simulink model "Drone2_simulink_old1"  (R2024b)
settings: Solver=ode1be  StartTime=0.0  StopTime=1200  FixedStep=0.001  MaxStep=0.001  MinStep=0.00095  RelTol=1e-3
undefined symbols (not defined in the file): DiscIntNeverNeededParam, Environment, Newton, Raphson, Sim3dSensor, Vehicle, X, Y, Z
libraries: sm_lib x2951, nesl_utility x76, slpidlib x25, simulink x4, eeGeneralControl x4, matrix_library x3, rllib x2, sim3dlib x2, uavsim3dlib x2, dspstat3 x1, SignalEditorBlockLib x1, sharedutil x1
(part 3 of 21)

== system Drone2_simulink_old1/Controller/RL System ==
  In1 : Inport
  In2 : Inport  Port=2
  In3 : Inport  Port=3
  In4 : Inport  Port=4
  In5 : Inport  Port=5
  In6 : Inport  Port=6
  In7 : Inport  Port=7
  In8 : Inport  Port=8
  In9 : Inport  Port=9
  In10 : Inport  Port=10
  isdone : Inport  Port=11
  Constant10 : Constant  Commented=on  Value=-4
  Constant11 : Constant  Commented=on  Value=0
  Demux : Demux  Commented=on  Outputs=2
  MATLAB Function2 : MATLAB Function  Commented=on  TreatAsAtomicUnit=on
  MATLAB Function3 : MATLAB Function  Commented=on  TreatAsAtomicUnit=on  mask{MaxPose=Vehicle.Syringe.Front.maxpos, MinPose=Vehicle.Syringe.Front.minpos, MaxVel=Vehicle.Syringe.MaxVelocity, Delta=0.0050, K=500.0}
  MATLAB Function4 : MATLAB Function  Commented=on  TreatAsAtomicUnit=on  mask{MaxPose=Vehicle.Syringe.Front.maxpos, MinPose=Vehicle.Syringe.Front.minpos, MaxVel=Vehicle.Syringe.MaxVelocity, Delta=0.0050}
  Mux : Mux  Commented=on  Inputs=2
  Mux1 : Mux  Commented=on  Inputs=12
  RL Agent : rllib/RL Agent  Commented=on  Agent=Controller.agent  ExternalActionAsInput=off  ProvideLastAction=off  ProvideCumRwd=off  TreatAsDirectFeedthrough=on  UseStrictObservationDataTypes=off
  Reshape : Reshape  Commented=on  OutputDimensionality=Customize
  front : Outport
  Back : Outport  Port=2
  wires:
  Mux1/1 -> MATLAB Function4/1(obs), RL Agent/1
  Constant10/1 -> Mux1/11, Mux/1
  Mux/1 -> MATLAB Function4/2(desired)
  In6/1 -> Mux1/6
  MATLAB Function4/1(reward) -> Reshape/1
  Constant11/1 -> Mux1/12, Mux/2
  In5/1 -> Mux1/5
  Reshape/1 -> RL Agent/2
  RL Agent/1 -> Demux/1
  In10/1 -> Mux1/10
  In4/1 -> Mux1/4
  In2/1 -> Mux1/2
  In3/1 -> Mux1/3
  isdone/1 -> RL Agent/3
  In7/1 -> Mux1/7
  In8/1 -> Mux1/8
  In9/1 -> Mux1/9
  Demux/1 -> front/1
  Demux/2 -> Back/1
  In1/1 -> Mux1/1

== system Drone2_simulink_old1/Controller/Underwater_Syringe_Actuation ==
  Z : Inport
  Z_desired : Inport  Port=2
  Vf_1 : Inport  Port=3
  Vf_2 : Inport  Port=4
  Theta : Inport  Port=5
  Theta Desired : Inport  Port=6
  Vb_prev : Inport  Port=7
  Derivative : Derivative  Commented=on
  Derivative1 : Derivative
  Discrete Derivative : simulink/Discrete/Discrete Derivative  Commented=on  gainval=1.0  ICPrevScaledInput=0.0  OutMin=[]  OutMax=[]  OutDataType=fixdt(1, 16)  OutScaling=2^-10  DoSatur=off
  Gain4 : Gain  Gain=0.5
  MATLAB Function1 : MATLAB Function  Commented=on  TreatAsAtomicUnit=on  mask{V_MIN=Vehicle.Syringe.Front.minpos, V_MAX=Vehicle.Syringe.Front.maxpos, V_DOT_MAX=0.012, HF=0.2, A=0, g=9.81, rho=1000, dt=0.001, Kp_pos=0.002, Kp_vel=0.002, Kr=0.005, EZDB=0.05, sigma=0.1, Ez_high=1, PLRate=0.0002, PKRate=0.05, ETDB=3}
      mask prompts: V_MIN "Min"; V_MAX "Max"; V_DOT_MAX "max rate"; HF "Half Length of drone"; A "Area of Syringe"; g "Gravity"; rho "Density"; dt "Sample Time"; Kp_pos "Learning Rate-Pose"; Kp_vel "Slow Learning Rate"; Kr "K_Rate"; EZDB "Error zone to reduce adaption"; sigma "Steady state error region"; Ez_high "mode switch region"; PLRate "Pitch Learning Rate"; PKRate "K_Rate"; ETDB "Error zone to reduce adaption"
  MATLAB Function7 : MATLAB Function  TreatAsAtomicUnit=on  mask{Min=Vehicle.Syringe.Front.minpos, Max=Vehicle.Syringe.Front.maxpos, HF=0.2, AS=0, G=9.81, RHO=1000, DT=0.001, DFRate=0.02, DMRate=0.002, DSRate=0.002, Dpanelty=0.005, EZDB=0.05, PLRate=0.0002, PKRate=0.05, ETDB=3}
      mask prompts: HF "Half Length of drone"; AS "Area of Syringe"; G "Gravity"; RHO "Density"; DT "Sample Time"; DFRate "Fast Learning rate with |e|>1"; DMRate "Medium Learning Rate"; DSRate "Slow Learning Rate"; Dpanelty "K_Rate"; EZDB "Error zone to reduce adaption"; PLRate "Pitch Learning Rate"; PKRate "K_Rate"; ETDB "Error zone to reduce adaption"
  PID Controller1 : slpidlib/PID Controller  Commented=on  Controller=PD  Form=Parallel  TimeDomain=Continuous-time  UseExternalTs=off  SampleTime=-1  IntegratorMethod=Forward Euler  FilterMethod=Forward Euler  ControllerParametersSource=internal  P=3500.0200194669353  I=843.52365195509  UseKiTs=on  D=26.9299392102605  UseExternalDerivativeSource=off  N=0.579906738639273  UseFilter=on  TunerSelectOption=Transfer Function Based (PID Tuner App)  InitialConditionSource=internal  InitialConditionForIntegrator=0  InitialConditionForFilter=0  DifferentiatorICPrevScaledInput=0  ExternalReset=none  TrackingMode=off  Kt=1  LimitOutput=on  SatLimitsSource=internal  UpperSaturationLimit=40  LowerSaturationLimit=0  LinearizeAsGain=on  AntiWindupMode=none  Kb=1  LimitIntegrator=off  UpperIntegratorSaturationLimit=inf  LowerIntegratorSaturationLimit=-inf  POutMin=[]  POutMax=[]  IOutMin=[]  IOutMax=[]  DOutMin=[]  DOutMax=[]  NOutMin=[]  NOutMax=[]  SumOutMin=[]  SumOutMax=[]  SaturationOutMin=[]  SaturationOutMax=[]  PParamMin=[]  PParamMax=[]  IParamMin=[]  IParamMax=[]  DParamMin=[]  DParamMax=[]  NParamMin=[]  NParamMax=[]  KbParamMin=[]  KbParamMax=[]  KtParamMin=[]  KtParamMax=[]  KbOutMin=[]  KbOutMax=[]  KtOutMin=[]  KtOutMax=[]  IntegratorOutMin=[]  IntegratorOutMax=[]  FilterOutMin=[]  FilterOutMax=[]  SumI1OutMin=[]  SumI1OutMax=[]  SumI2OutMin=[]  SumI2OutMax=[]  SumI3OutMin=[]  SumI3OutMax=[]  SumI4OutMin=[]  SumI4OutMax=[]  SumDOutMin=[]  SumDOutMax=[]  DifferentiatorOutMin=[]  DifferentiatorOutMax=[]  FilterDiffOutCoefMin=[]  FilterDiffOutCoefMax=[]  ReciprocalOutMin=[]  ReciprocalOutMax=[]  SumDenOutMin=[]  SumDenOutMax=[]  SumNumOutMin=[]  SumNumOutMax=[]  DivideOutMin=[]  DivideOutMax=[]  UdiffTsProdOutMin=[]  UdiffTsProdOutMax=[]  NTsProdOutMin=[]  NTsProdOutMax=[]  UintegralTsProdOutMin=[]  UintegralTsProdOutMax=[]  UngainTsProdOutMin=[]  UngainTsProdOutMax=[]  ClampingZeroOutDataTypeStr=Inherit: Inherit via back propagation  ClampingZeroOutMin=[]  ClampingZeroOutMax=[]  FilterDenConstantOutDataTypeStr=Inherit: Inherit via back propagation  FilterDenConstantOutMin=[]  FilterDenConstantOutMax=[]  PCopyOutDataTypeStr=Inherit: Inherit via back propagation  PCopyOutMin=[]  PCopyOutMax=[]  NCopyOutDataTypeStr=Inherit: Inherit via back propagation  NCopyOutMin=[]  NCopyOutMax=[]  IntegratorContinuousStateAttributes=''  IntegratorStateMustResolveToSignalObject=off  IntegratorRTWStateStorageClass=Auto  FilterContinuousStateAttributes=''  FilterStateMustResolveToSignalObject=off  FilterRTWStateStorageClass=Auto  ParallelPVariant=InternalParameters  IdealPVariant=Disabled  IVariant=Disabled  DVariant=InternalParameters  IntegratorVariant=Disabled  SatVariant=Enabled  AWVariant=Disabled  PCopyVariant=Disabled  TRVariant=Disabled  FdbkBlocksVariant=Forward  IdealPFdbkVariant=Disabled  SatFdbkVariant=Disabled  DerivativeFilterVariant=ContFilter  NVariant=InternalParameters  NCopyVariant=Disabled  FilterICVariant=InternalICsFilter  IntegratorICVariant=Disabled  ExternalResetVariant=Disabled  TRSumVariant=Passthrough  SumFdbkVariant=Disabled  SumVariant=Sum_PD  TsampFilterVariant=InternalTs  TsampNgainVariant=Passthrough  TsampIntegralVariant=Disabled_SignalSpec  ExternalSaturationOutDataTypeStr=Inherit: Same as second input  DerivativeSourceVariant=ErrorSignal
  PID Controller2 : slpidlib/PID Controller  Commented=on  Controller=PD  Form=Parallel  TimeDomain=Continuous-time  UseExternalTs=off  SampleTime=-1  IntegratorMethod=Forward Euler  FilterMethod=Forward Euler  ControllerParametersSource=internal  P=3744.13110896654  I=964.677966952311  UseKiTs=on  D=30  UseExternalDerivativeSource=off  N=0.58  UseFilter=on  TunerSelectOption=Transfer Function Based (PID Tuner App)  InitialConditionSource=internal  InitialConditionForIntegrator=0  InitialConditionForFilter=0  DifferentiatorICPrevScaledInput=0  ExternalReset=none  TrackingMode=off  Kt=1  LimitOutput=on  SatLimitsSource=internal  UpperSaturationLimit=40  LowerSaturationLimit=0  LinearizeAsGain=on  AntiWindupMode=none  Kb=1  LimitIntegrator=off  UpperIntegratorSaturationLimit=inf  LowerIntegratorSaturationLimit=-inf  POutMin=[]  POutMax=[]  IOutMin=[]  IOutMax=[]  DOutMin=[]  DOutMax=[]  NOutMin=[]  NOutMax=[]  SumOutMin=[]  SumOutMax=[]  SaturationOutMin=[]  SaturationOutMax=[]  PParamMin=[]  PParamMax=[]  IParamMin=[]  IParamMax=[]  DParamMin=[]  DParamMax=[]  NParamMin=[]  NParamMax=[]  KbParamMin=[]  KbParamMax=[]  KtParamMin=[]  KtParamMax=[]  KbOutMin=[]  KbOutMax=[]  KtOutMin=[]  KtOutMax=[]  IntegratorOutMin=[]  IntegratorOutMax=[]  FilterOutMin=[]  FilterOutMax=[]  SumI1OutMin=[]  SumI1OutMax=[]  SumI2OutMin=[]  SumI2OutMax=[]  SumI3OutMin=[]  SumI3OutMax=[]  SumI4OutMin=[]  SumI4OutMax=[]  SumDOutMin=[]  SumDOutMax=[]  DifferentiatorOutMin=[]  DifferentiatorOutMax=[]  FilterDiffOutCoefMin=[]  FilterDiffOutCoefMax=[]  ReciprocalOutMin=[]  ReciprocalOutMax=[]  SumDenOutMin=[]  SumDenOutMax=[]  SumNumOutMin=[]  SumNumOutMax=[]  DivideOutMin=[]  DivideOutMax=[]  UdiffTsProdOutMin=[]  UdiffTsProdOutMax=[]  NTsProdOutMin=[]  NTsProdOutMax=[]  UintegralTsProdOutMin=[]  UintegralTsProdOutMax=[]  UngainTsProdOutMin=[]  UngainTsProdOutMax=[]  ClampingZeroOutDataTypeStr=Inherit: Inherit via back propagation  ClampingZeroOutMin=[]  ClampingZeroOutMax=[]  FilterDenConstantOutDataTypeStr=Inherit: Inherit via back propagation  FilterDenConstantOutMin=[]  FilterDenConstantOutMax=[]  PCopyOutDataTypeStr=Inherit: Inherit via back propagation  PCopyOutMin=[]  PCopyOutMax=[]  NCopyOutDataTypeStr=Inherit: Inherit via back propagation  NCopyOutMin=[]  NCopyOutMax=[]  IntegratorContinuousStateAttributes=''  IntegratorStateMustResolveToSignalObject=off  IntegratorRTWStateStorageClass=Auto  FilterContinuousStateAttributes=''  FilterStateMustResolveToSignalObject=off  FilterRTWStateStorageClass=Auto  ParallelPVariant=InternalParameters  IdealPVariant=Disabled  IVariant=Disabled  DVariant=InternalParameters  IntegratorVariant=Disabled  SatVariant=Enabled  AWVariant=Disabled  PCopyVariant=Disabled  TRVariant=Disabled  FdbkBlocksVariant=Forward  IdealPFdbkVariant=Disabled  SatFdbkVariant=Disabled  DerivativeFilterVariant=ContFilter  NVariant=InternalParameters  NCopyVariant=Disabled  FilterICVariant=InternalICsFilter  IntegratorICVariant=Disabled  ExternalResetVariant=Disabled  TRSumVariant=Passthrough  SumFdbkVariant=Disabled  SumVariant=Sum_PD  TsampFilterVariant=InternalTs  TsampNgainVariant=Passthrough  TsampIntegralVariant=Disabled_SignalSpec  ExternalSaturationOutDataTypeStr=Inherit: Same as second input  DerivativeSourceVariant=ErrorSignal
  PID Controller4 : slpidlib/PID Controller  Controller=PD  Form=Parallel  TimeDomain=Continuous-time  UseExternalTs=off  SampleTime=-1  IntegratorMethod=Forward Euler  FilterMethod=Forward Euler  ControllerParametersSource=internal  P=8  I=0  UseKiTs=on  D=0.5  UseExternalDerivativeSource=off  N=20  UseFilter=on  TunerSelectOption=Transfer Function Based (PID Tuner App)  InitialConditionSource=internal  InitialConditionForIntegrator=0  InitialConditionForFilter=0  DifferentiatorICPrevScaledInput=0  ExternalReset=none  TrackingMode=off  Kt=1  LimitOutput=off  SatLimitsSource=internal  UpperSaturationLimit=Vehicle.Syringe.Thrustlim  LowerSaturationLimit=-Vehicle.Syringe.Thrustlim  LinearizeAsGain=on  AntiWindupMode=none  Kb=1  LimitIntegrator=off  UpperIntegratorSaturationLimit=inf  LowerIntegratorSaturationLimit=-inf  POutMin=[]  POutMax=[]  IOutMin=[]  IOutMax=[]  DOutMin=[]  DOutMax=[]  NOutMin=[]  NOutMax=[]  SumOutMin=[]  SumOutMax=[]  SaturationOutMin=[]  SaturationOutMax=[]  PParamMin=[]  PParamMax=[]  IParamMin=[]  IParamMax=[]  DParamMin=[]  DParamMax=[]  NParamMin=[]  NParamMax=[]  KbParamMin=[]  KbParamMax=[]  KtParamMin=[]  KtParamMax=[]  KbOutMin=[]  KbOutMax=[]  KtOutMin=[]  KtOutMax=[]  IntegratorOutMin=[]  IntegratorOutMax=[]  FilterOutMin=[]  FilterOutMax=[]  SumI1OutMin=[]  SumI1OutMax=[]  SumI2OutMin=[]  SumI2OutMax=[]  SumI3OutMin=[]  SumI3OutMax=[]  SumI4OutMin=[]  SumI4OutMax=[]  SumDOutMin=[]  SumDOutMax=[]  DifferentiatorOutMin=[]  DifferentiatorOutMax=[]  FilterDiffOutCoefMin=[]  FilterDiffOutCoefMax=[]  ReciprocalOutMin=[]  ReciprocalOutMax=[]  SumDenOutMin=[]  SumDenOutMax=[]  SumNumOutMin=[]  SumNumOutMax=[]  DivideOutMin=[]  DivideOutMax=[]  UdiffTsProdOutMin=[]  UdiffTsProdOutMax=[]  NTsProdOutMin=[]  NTsProdOutMax=[]  UintegralTsProdOutMin=[]  UintegralTsProdOutMax=[]  UngainTsProdOutMin=[]  UngainTsProdOutMax=[]  ClampingZeroOutDataTypeStr=Inherit: Inherit via back propagation  ClampingZeroOutMin=[]  ClampingZeroOutMax=[]  FilterDenConstantOutDataTypeStr=Inherit: Inherit via back propagation  FilterDenConstantOutMin=[]  FilterDenConstantOutMax=[]  PCopyOutDataTypeStr=Inherit: Inherit via back propagation  PCopyOutMin=[]  PCopyOutMax=[]  NCopyOutDataTypeStr=Inherit: Inherit via back propagation  NCopyOutMin=[]  NCopyOutMax=[]  IntegratorContinuousStateAttributes=''  IntegratorStateMustResolveToSignalObject=off  IntegratorRTWStateStorageClass=Auto  FilterContinuousStateAttributes=''  FilterStateMustResolveToSignalObject=off  FilterRTWStateStorageClass=Auto  ParallelPVariant=InternalParameters  IdealPVariant=Disabled  IVariant=Disabled  DVariant=InternalParameters  IntegratorVariant=Disabled  SatVariant=Disabled  AWVariant=Disabled  PCopyVariant=Disabled  TRVariant=Disabled  FdbkBlocksVariant=Forward  IdealPFdbkVariant=Disabled  SatFdbkVariant=Disabled  DerivativeFilterVariant=ContFilter  NVariant=InternalParameters  NCopyVariant=Disabled  FilterICVariant=InternalICsFilter  IntegratorICVariant=Disabled  ExternalResetVariant=Disabled  TRSumVariant=Passthrough  SumFdbkVariant=Disabled  SumVariant=Sum_PD  TsampFilterVariant=InternalTs  TsampNgainVariant=Passthrough  TsampIntegralVariant=Disabled_SignalSpec  ExternalSaturationOutDataTypeStr=Inherit: Same as second input  DerivativeSourceVariant=ErrorSignal
  PID Controller5 : slpidlib/PID Controller  Controller=PD  Form=Parallel  TimeDomain=Continuous-time  UseExternalTs=off  SampleTime=-1  IntegratorMethod=Forward Euler  FilterMethod=Forward Euler  ControllerParametersSource=internal  P=4  I=0  UseKiTs=on  D=0.5  UseExternalDerivativeSource=off  N=100  UseFilter=on  TunerSelectOption=Transfer Function Based (PID Tuner App)  InitialConditionSource=internal  InitialConditionForIntegrator=0  InitialConditionForFilter=0  DifferentiatorICPrevScaledInput=0  ExternalReset=none  TrackingMode=off  Kt=1  LimitOutput=off  SatLimitsSource=internal  UpperSaturationLimit=Vehicle.Syringe.Thrustlim  LowerSaturationLimit=-Vehicle.Syringe.Thrustlim  LinearizeAsGain=on  AntiWindupMode=none  Kb=1  LimitIntegrator=off  UpperIntegratorSaturationLimit=inf  LowerIntegratorSaturationLimit=-inf  POutMin=[]  POutMax=[]  IOutMin=[]  IOutMax=[]  DOutMin=[]  DOutMax=[]  NOutMin=[]  NOutMax=[]  SumOutMin=[]  SumOutMax=[]  SaturationOutMin=[]  SaturationOutMax=[]  PParamMin=[]  PParamMax=[]  IParamMin=[]  IParamMax=[]  DParamMin=[]  DParamMax=[]  NParamMin=[]  NParamMax=[]  KbParamMin=[]  KbParamMax=[]  KtParamMin=[]  KtParamMax=[]  KbOutMin=[]  KbOutMax=[]  KtOutMin=[]  KtOutMax=[]  IntegratorOutMin=[]  IntegratorOutMax=[]  FilterOutMin=[]  FilterOutMax=[]  SumI1OutMin=[]  SumI1OutMax=[]  SumI2OutMin=[]  SumI2OutMax=[]  SumI3OutMin=[]  SumI3OutMax=[]  SumI4OutMin=[]  SumI4OutMax=[]  SumDOutMin=[]  SumDOutMax=[]  DifferentiatorOutMin=[]  DifferentiatorOutMax=[]  FilterDiffOutCoefMin=[]  FilterDiffOutCoefMax=[]  ReciprocalOutMin=[]  ReciprocalOutMax=[]  SumDenOutMin=[]  SumDenOutMax=[]  SumNumOutMin=[]  SumNumOutMax=[]  DivideOutMin=[]  DivideOutMax=[]  UdiffTsProdOutMin=[]  UdiffTsProdOutMax=[]  NTsProdOutMin=[]  NTsProdOutMax=[]  UintegralTsProdOutMin=[]  UintegralTsProdOutMax=[]  UngainTsProdOutMin=[]  UngainTsProdOutMax=[]  ClampingZeroOutDataTypeStr=Inherit: Inherit via back propagation  ClampingZeroOutMin=[]  ClampingZeroOutMax=[]  FilterDenConstantOutDataTypeStr=Inherit: Inherit via back propagation  FilterDenConstantOutMin=[]  FilterDenConstantOutMax=[]  PCopyOutDataTypeStr=Inherit: Inherit via back propagation  PCopyOutMin=[]  PCopyOutMax=[]  NCopyOutDataTypeStr=Inherit: Inherit via back propagation  NCopyOutMin=[]  NCopyOutMax=[]  IntegratorContinuousStateAttributes=''  IntegratorStateMustResolveToSignalObject=off  IntegratorRTWStateStorageClass=Auto  FilterContinuousStateAttributes=''  FilterStateMustResolveToSignalObject=off  FilterRTWStateStorageClass=Auto  ParallelPVariant=InternalParameters  IdealPVariant=Disabled  IVariant=Disabled  DVariant=InternalParameters  IntegratorVariant=Disabled  SatVariant=Disabled  AWVariant=Disabled  PCopyVariant=Disabled  TRVariant=Disabled  FdbkBlocksVariant=Forward  IdealPFdbkVariant=Disabled  SatFdbkVariant=Disabled  DerivativeFilterVariant=ContFilter  NVariant=InternalParameters  NCopyVariant=Disabled  FilterICVariant=InternalICsFilter  IntegratorICVariant=Disabled  ExternalResetVariant=Disabled  TRSumVariant=Passthrough  SumFdbkVariant=Disabled  SumVariant=Sum_PD  TsampFilterVariant=InternalTs  TsampNgainVariant=Passthrough  TsampIntegralVariant=Disabled_SignalSpec  ExternalSaturationOutDataTypeStr=Inherit: Same as second input  DerivativeSourceVariant=ErrorSignal
  PID Controller6 : slpidlib/PID Controller  Controller=PD  Form=Parallel  TimeDomain=Continuous-time  UseExternalTs=off  SampleTime=-1  IntegratorMethod=Forward Euler  FilterMethod=Forward Euler  ControllerParametersSource=internal  P=3500  I=843.52365195509  UseKiTs=on  D=30  UseExternalDerivativeSource=off  N=1  UseFilter=on  TunerSelectOption=Transfer Function Based (PID Tuner App)  InitialConditionSource=internal  InitialConditionForIntegrator=0  InitialConditionForFilter=0  DifferentiatorICPrevScaledInput=0  ExternalReset=none  TrackingMode=off  Kt=1  LimitOutput=on  SatLimitsSource=internal  UpperSaturationLimit=40  LowerSaturationLimit=0  LinearizeAsGain=on  AntiWindupMode=none  Kb=1  LimitIntegrator=off  UpperIntegratorSaturationLimit=inf  LowerIntegratorSaturationLimit=-inf  POutMin=[]  POutMax=[]  IOutMin=[]  IOutMax=[]  DOutMin=[]  DOutMax=[]  NOutMin=[]  NOutMax=[]  SumOutMin=[]  SumOutMax=[]  SaturationOutMin=[]  SaturationOutMax=[]  PParamMin=[]  PParamMax=[]  IParamMin=[]  IParamMax=[]  DParamMin=[]  DParamMax=[]  NParamMin=[]  NParamMax=[]  KbParamMin=[]  KbParamMax=[]  KtParamMin=[]  KtParamMax=[]  KbOutMin=[]  KbOutMax=[]  KtOutMin=[]  KtOutMax=[]  IntegratorOutMin=[]  IntegratorOutMax=[]  FilterOutMin=[]  FilterOutMax=[]  SumI1OutMin=[]  SumI1OutMax=[]  SumI2OutMin=[]  SumI2OutMax=[]  SumI3OutMin=[]  SumI3OutMax=[]  SumI4OutMin=[]  SumI4OutMax=[]  SumDOutMin=[]  SumDOutMax=[]  DifferentiatorOutMin=[]  DifferentiatorOutMax=[]  FilterDiffOutCoefMin=[]  FilterDiffOutCoefMax=[]  ReciprocalOutMin=[]  ReciprocalOutMax=[]  SumDenOutMin=[]  SumDenOutMax=[]  SumNumOutMin=[]  SumNumOutMax=[]  DivideOutMin=[]  DivideOutMax=[]  UdiffTsProdOutMin=[]  UdiffTsProdOutMax=[]  NTsProdOutMin=[]  NTsProdOutMax=[]  UintegralTsProdOutMin=[]  UintegralTsProdOutMax=[]  UngainTsProdOutMin=[]  UngainTsProdOutMax=[]  ClampingZeroOutDataTypeStr=Inherit: Inherit via back propagation  ClampingZeroOutMin=[]  ClampingZeroOutMax=[]  FilterDenConstantOutDataTypeStr=Inherit: Inherit via back propagation  FilterDenConstantOutMin=[]  FilterDenConstantOutMax=[]  PCopyOutDataTypeStr=Inherit: Inherit via back propagation  PCopyOutMin=[]  PCopyOutMax=[]  NCopyOutDataTypeStr=Inherit: Inherit via back propagation  NCopyOutMin=[]  NCopyOutMax=[]  IntegratorContinuousStateAttributes=''  IntegratorStateMustResolveToSignalObject=off  IntegratorRTWStateStorageClass=Auto  FilterContinuousStateAttributes=''  FilterStateMustResolveToSignalObject=off  FilterRTWStateStorageClass=Auto  ParallelPVariant=InternalParameters  IdealPVariant=Disabled  IVariant=Disabled  DVariant=InternalParameters  IntegratorVariant=Disabled  SatVariant=Enabled  AWVariant=Disabled  PCopyVariant=Disabled  TRVariant=Disabled  FdbkBlocksVariant=Forward  IdealPFdbkVariant=Disabled  SatFdbkVariant=Disabled  DerivativeFilterVariant=ContFilter  NVariant=InternalParameters  NCopyVariant=Disabled  FilterICVariant=InternalICsFilter  IntegratorICVariant=Disabled  ExternalResetVariant=Disabled  TRSumVariant=Passthrough  SumFdbkVariant=Disabled  SumVariant=Sum_PD  TsampFilterVariant=InternalTs  TsampNgainVariant=Passthrough  TsampIntegralVariant=Disabled_SignalSpec  ExternalSaturationOutDataTypeStr=Inherit: Same as second input  DerivativeSourceVariant=ErrorSignal
  PID Controller7 : slpidlib/PID Controller  Controller=PD  Form=Parallel  TimeDomain=Continuous-time  UseExternalTs=off  SampleTime=-1  IntegratorMethod=Forward Euler  FilterMethod=Forward Euler  ControllerParametersSource=internal  P=3750  I=964.677966952311  UseKiTs=on  D=30  UseExternalDerivativeSource=off  N=1  UseFilter=on  TunerSelectOption=Transfer Function Based (PID Tuner App)  InitialConditionSource=internal  InitialConditionForIntegrator=0  InitialConditionForFilter=0  DifferentiatorICPrevScaledInput=0  ExternalReset=none  TrackingMode=off  Kt=1  LimitOutput=on  SatLimitsSource=internal  UpperSaturationLimit=40  LowerSaturationLimit=0  LinearizeAsGain=on  AntiWindupMode=none  Kb=1  LimitIntegrator=off  UpperIntegratorSaturationLimit=inf  LowerIntegratorSaturationLimit=-inf  POutMin=[]  POutMax=[]  IOutMin=[]  IOutMax=[]  DOutMin=[]  DOutMax=[]  NOutMin=[]  NOutMax=[]  SumOutMin=[]  SumOutMax=[]  SaturationOutMin=[]  SaturationOutMax=[]  PParamMin=[]  PParamMax=[]  IParamMin=[]  IParamMax=[]  DParamMin=[]  DParamMax=[]  NParamMin=[]  NParamMax=[]  KbParamMin=[]  KbParamMax=[]  KtParamMin=[]  KtParamMax=[]  KbOutMin=[]  KbOutMax=[]  KtOutMin=[]  KtOutMax=[]  IntegratorOutMin=[]  IntegratorOutMax=[]  FilterOutMin=[]  FilterOutMax=[]  SumI1OutMin=[]  SumI1OutMax=[]  SumI2OutMin=[]  SumI2OutMax=[]  SumI3OutMin=[]  SumI3OutMax=[]  SumI4OutMin=[]  SumI4OutMax=[]  SumDOutMin=[]  SumDOutMax=[]  DifferentiatorOutMin=[]  DifferentiatorOutMax=[]  FilterDiffOutCoefMin=[]  FilterDiffOutCoefMax=[]  ReciprocalOutMin=[]  ReciprocalOutMax=[]  SumDenOutMin=[]  SumDenOutMax=[]  SumNumOutMin=[]  SumNumOutMax=[]  DivideOutMin=[]  DivideOutMax=[]  UdiffTsProdOutMin=[]  UdiffTsProdOutMax=[]  NTsProdOutMin=[]  NTsProdOutMax=[]  UintegralTsProdOutMin=[]  UintegralTsProdOutMax=[]  UngainTsProdOutMin=[]  UngainTsProdOutMax=[]  ClampingZeroOutDataTypeStr=Inherit: Inherit via back propagation  ClampingZeroOutMin=[]  ClampingZeroOutMax=[]  FilterDenConstantOutDataTypeStr=Inherit: Inherit via back propagation  FilterDenConstantOutMin=[]  FilterDenConstantOutMax=[]  PCopyOutDataTypeStr=Inherit: Inherit via back propagation  PCopyOutMin=[]  PCopyOutMax=[]  NCopyOutDataTypeStr=Inherit: Inherit via back propagation  NCopyOutMin=[]  NCopyOutMax=[]  IntegratorContinuousStateAttributes=''  IntegratorStateMustResolveToSignalObject=off  IntegratorRTWStateStorageClass=Auto  FilterContinuousStateAttributes=''  FilterStateMustResolveToSignalObject=off  FilterRTWStateStorageClass=Auto  ParallelPVariant=InternalParameters  IdealPVariant=Disabled  IVariant=Disabled  DVariant=InternalParameters  IntegratorVariant=Disabled  SatVariant=Enabled  AWVariant=Disabled  PCopyVariant=Disabled  TRVariant=Disabled  FdbkBlocksVariant=Forward  IdealPFdbkVariant=Disabled  SatFdbkVariant=Disabled  DerivativeFilterVariant=ContFilter  NVariant=InternalParameters  NCopyVariant=Disabled  FilterICVariant=InternalICsFilter  IntegratorICVariant=Disabled  ExternalResetVariant=Disabled  TRSumVariant=Passthrough  SumFdbkVariant=Disabled  SumVariant=Sum_PD  TsampFilterVariant=InternalTs  TsampNgainVariant=Passthrough  TsampIntegralVariant=Disabled_SignalSpec  ExternalSaturationOutDataTypeStr=Inherit: Same as second input  DerivativeSourceVariant=ErrorSignal
  PID Controller8 : slpidlib/PID Controller  Commented=on  Controller=PID  Form=Parallel  TimeDomain=Continuous-time  UseExternalTs=off  SampleTime=-1  IntegratorMethod=Forward Euler  FilterMethod=Forward Euler  ControllerParametersSource=internal  P=44.1440048797783  I=843.52365195509  UseKiTs=on  D=0  UseExternalDerivativeSource=off  N=100  UseFilter=on  TunerSelectOption=Transfer Function Based (PID Tuner App)  InitialConditionSource=internal  InitialConditionForIntegrator=0  InitialConditionForFilter=0  DifferentiatorICPrevScaledInput=0  ExternalReset=none  TrackingMode=off  Kt=1  LimitOutput=on  SatLimitsSource=internal  UpperSaturationLimit=40  LowerSaturationLimit=0  LinearizeAsGain=on  AntiWindupMode=none  Kb=1  LimitIntegrator=off  UpperIntegratorSaturationLimit=inf  LowerIntegratorSaturationLimit=-inf  POutMin=[]  POutMax=[]  IOutMin=[]  IOutMax=[]  DOutMin=[]  DOutMax=[]  NOutMin=[]  NOutMax=[]  SumOutMin=[]  SumOutMax=[]  SaturationOutMin=[]  SaturationOutMax=[]  PParamMin=[]  PParamMax=[]  IParamMin=[]  IParamMax=[]  DParamMin=[]  DParamMax=[]  NParamMin=[]  NParamMax=[]  KbParamMin=[]  KbParamMax=[]  KtParamMin=[]  KtParamMax=[]  KbOutMin=[]  KbOutMax=[]  KtOutMin=[]  KtOutMax=[]  IntegratorOutMin=[]  IntegratorOutMax=[]  FilterOutMin=[]  FilterOutMax=[]  SumI1OutMin=[]  SumI1OutMax=[]  SumI2OutMin=[]  SumI2OutMax=[]  SumI3OutMin=[]  SumI3OutMax=[]  SumI4OutMin=[]  SumI4OutMax=[]  SumDOutMin=[]  SumDOutMax=[]  DifferentiatorOutMin=[]  DifferentiatorOutMax=[]  FilterDiffOutCoefMin=[]  FilterDiffOutCoefMax=[]  ReciprocalOutMin=[]  ReciprocalOutMax=[]  SumDenOutMin=[]  SumDenOutMax=[]  SumNumOutMin=[]  SumNumOutMax=[]  DivideOutMin=[]  DivideOutMax=[]  UdiffTsProdOutMin=[]  UdiffTsProdOutMax=[]  NTsProdOutMin=[]  NTsProdOutMax=[]  UintegralTsProdOutMin=[]  UintegralTsProdOutMax=[]  UngainTsProdOutMin=[]  UngainTsProdOutMax=[]  ClampingZeroOutDataTypeStr=Inherit: Inherit via back propagation  ClampingZeroOutMin=[]  ClampingZeroOutMax=[]  FilterDenConstantOutDataTypeStr=Inherit: Inherit via back propagation  FilterDenConstantOutMin=[]  FilterDenConstantOutMax=[]  PCopyOutDataTypeStr=Inherit: Inherit via back propagation  PCopyOutMin=[]  PCopyOutMax=[]  NCopyOutDataTypeStr=Inherit: Inherit via back propagation  NCopyOutMin=[]  NCopyOutMax=[]  IntegratorContinuousStateAttributes=''  IntegratorStateMustResolveToSignalObject=off  IntegratorRTWStateStorageClass=Auto  FilterContinuousStateAttributes=''  FilterStateMustResolveToSignalObject=off  FilterRTWStateStorageClass=Auto  ParallelPVariant=InternalParameters  IdealPVariant=Disabled  IVariant=InternalParameters  DVariant=InternalParameters  IntegratorVariant=Continuous  SatVariant=Enabled  AWVariant=Passthrough  PCopyVariant=Disabled  TRVariant=Disabled  FdbkBlocksVariant=Forward  IdealPFdbkVariant=Disabled  SatFdbkVariant=Disabled  DerivativeFilterVariant=ContFilter  NVariant=InternalParameters  NCopyVariant=Disabled  FilterICVariant=InternalICsFilter  IntegratorICVariant=InternalICs  ExternalResetVariant=Disabled  TRSumVariant=Passthrough  SumFdbkVariant=Disabled  SumVariant=Sum_PID  TsampFilterVariant=InternalTs  TsampNgainVariant=Passthrough  TsampIntegralVariant=Disabled_SignalSpec  ExternalSaturationOutDataTypeStr=Inherit: Same as second input  DerivativeSourceVariant=ErrorSignal
  PID1 : Scope  NumInputPorts=2
  PID3 : Scope  NumInputPorts=2
  Scope3 : Scope  NumInputPorts=2
  Scope5 : Scope  NumInputPorts=2
  Subtract6 : Sum  Inputs=+-
  Subtract7 : Sum  Inputs=+-
  Subtract8 : Sum  Inputs=-+
  Subtract9 : Sum  Inputs=+-
  Sum : Sum  Inputs=|++
  desired : Scope  NumInputPorts=2
  error : Scope  NumInputPorts=2
  Front_Syringe : Outport
  Back_Syringe : Outport  Port=2
  wires:
  Subtract9/1 -> error/2, PID Controller7/1  "e_bpos"
  Vf_1/1 -> Sum/1
  Vf_2/1 -> Sum/2
  MATLAB Function7/2(Vb_cmd) -> Scope3/2
  Subtract8/1 -> error/1, PID Controller6/1  "error in FS"
  Z/1 -> MATLAB Function1/2(Z), MATLAB Function7/2(Z), Subtract6/1
  Sum/1 -> Gain4/1
  Theta/1 -> Subtract7/1
  Theta Desired/1 -> Subtract7/2
  Subtract7/1 -> Scope5/2, MATLAB Function7/7(etheta), Derivative1/1, PID Controller5/1  "etheta"
  Gain4/1 -> Subtract8/1, MATLAB Function7/9(Vf_prev)
  PID Controller4/1 -> MATLAB Function1/1(F_b), MATLAB Function7/3(F_b), PID1/1  "Freq"
  Derivative1/1 -> MATLAB Function7/8(etheta_dot)
  MATLAB Function7/1(Vf_cmd) -> Scope3/1
  PID Controller5/1 -> MATLAB Function7/4(tb), PID1/2  "t_req"
  Vb_prev/1 -> Subtract9/2, MATLAB Function7/10(Vb_prev)
  MATLAB Function7/3(Vf_trim_hat) -> Subtract8/2, desired/1
  MATLAB Function7/4(Vb_trim_hat) -> Subtract9/1, desired/2
  PID Controller6/1 -> PID3/1, Front_Syringe/1
  PID Controller7/1 -> PID3/2, Back_Syringe/1
  Z_desired/1 -> MATLAB Function7/1(Z_desired), MATLAB Function1/3(Zdesired), Subtract6/2
  Subtract6/1 -> Discrete Derivative/1, MATLAB Function1/5(ez_dot), MATLAB Function7/6(ez_dot), Scope5/1, MATLAB Function1/4(ez), MATLAB Function7/5(ez), PID Controller4/1

== system Drone2_simulink_old1/Controller (STA-Based)/Desired ==
  note: $\text{Sine wave} = \text{startpose(3)}+0.5*sin\left(\frac{2*pi}{200}t\right)$
  note: $\text{Ramp} = \text{startpose(3)}-0.005t \qquad 0<t<400$
  Add2 : Sum
  Constant8 : Constant  Value=Vehicle.Target.Desired
  Manual Switch : ManualSwitch
  Manual Switch1 : ManualSwitch  CurrentSetting=0
  Mux : Mux  Inputs=2
  Ramp : simulink/Sources/Ramp  slope=-0.005  start=0  InitialOutput=Vehicle.InitCond.position(3)
  Ramp1 : simulink/Sources/Ramp  slope=0.005  start=400  InitialOutput=Vehicle.InitCond.position(3)
  Selector : Selector  InputPortWidth=6  IndexOptions=Index vector (dialog)  Indices=[2 3 4 5 6]  OutputSizes=1
  Sine Wave : Sin  Amplitude=0.5  Bias=Vehicle.InitCond.position(3)  Frequency=2*pi/200  SampleTime=0
  Zd : Outport
  wires:
  Ramp1/1 -> Add2/2
  Add2/1 -> Manual Switch/2
  Sine Wave/1 -> Manual Switch/1
  Ramp/1 -> Add2/1
  Constant8/1 -> Selector/1, Manual Switch1/1
  Manual Switch/1 -> [zsec]
  [zsec] -> Mux/1
  Selector/1 -> Mux/2
  Mux/1 -> Manual Switch1/2
  Manual Switch1/1 -> Zd/1

== system Drone2_simulink_old1/Controller (STA-Based)/RL System ==
  In1 : Inport
  In2 : Inport  Port=2
  In3 : Inport  Port=3
  In4 : Inport  Port=4
  In5 : Inport  Port=5
  In6 : Inport  Port=6
  In7 : Inport  Port=7
  In8 : Inport  Port=8
  In9 : Inport  Port=9
  In10 : Inport  Port=10
  isdone : Inport  Port=11
  Constant10 : Constant  Commented=on  Value=-4
  Constant11 : Constant  Commented=on  Value=0
  Demux : Demux  Commented=on  Outputs=2
  MATLAB Function2 : MATLAB Function  Commented=on  TreatAsAtomicUnit=on
  MATLAB Function3 : MATLAB Function  Commented=on  TreatAsAtomicUnit=on  mask{MaxPose=Vehicle.Syringe.Front.maxpos, MinPose=Vehicle.Syringe.Front.minpos, MaxVel=Vehicle.Syringe.MaxVelocity, Delta=0.0050, K=500.0}
  MATLAB Function4 : MATLAB Function  Commented=on  TreatAsAtomicUnit=on  mask{MaxPose=Vehicle.Syringe.Front.maxpos, MinPose=Vehicle.Syringe.Front.minpos, MaxVel=Vehicle.Syringe.MaxVelocity, Delta=0.0050}
  Mux : Mux  Commented=on  Inputs=2
  Mux1 : Mux  Commented=on  Inputs=12
  RL Agent : rllib/RL Agent  Commented=on  Agent=Controller.agent  ExternalActionAsInput=off  ProvideLastAction=off  ProvideCumRwd=off  TreatAsDirectFeedthrough=on  UseStrictObservationDataTypes=off
  Reshape : Reshape  Commented=on  OutputDimensionality=Customize
  front : Outport
  Back : Outport  Port=2
  wires:
  In1/1 -> Mux1/1
  Demux/2 -> Back/1
  Demux/1 -> front/1
  In9/1 -> Mux1/9
  In8/1 -> Mux1/8
  In7/1 -> Mux1/7
  isdone/1 -> RL Agent/3
  In3/1 -> Mux1/3
  In2/1 -> Mux1/2
  In4/1 -> Mux1/4
  In10/1 -> Mux1/10
  RL Agent/1 -> Demux/1
  Reshape/1 -> RL Agent/2
  In5/1 -> Mux1/5
  Constant11/1 -> Mux/2, Mux1/12
  MATLAB Function4/1(reward) -> Reshape/1
  In6/1 -> Mux1/6
  Mux/1 -> MATLAB Function4/2(desired)
  Constant10/1 -> Mux/1, Mux1/11
  Mux1/1 -> RL Agent/1, MATLAB Function4/1(obs)

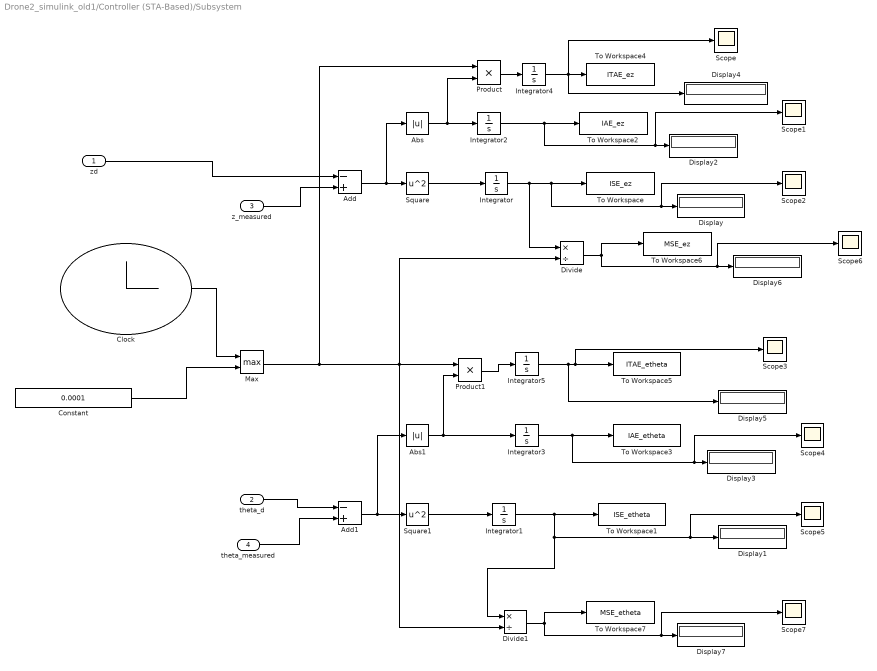
== system Drone2_simulink_old1/Controller (STA-Based)/Subsystem ==
  zd : Inport
  theta_d : Inport  Port=2
  z_measured : Inport  Port=3
  theta_measured : Inport  Port=4
  Abs : Abs  SaturateOnIntegerOverflow=off
  Abs1 : Abs  SaturateOnIntegerOverflow=off
  Add : Sum  Inputs=-+
  Add1 : Sum  Inputs=-+
  Clock : Clock
  Constant : Constant  Value=0.0001
  Display{,1..7} (8 alike) : Display
  Divide : Product  Inputs=*/
  Divide1 : Product  Inputs=*/
  Integrator{,1..5} (6 alike) : Integrator
  Max : MinMax  Function=max  Inputs=2
  Product : Product
  Product1 : Product
  Scope{,1..7} (8 alike) : Scope
  Square : Math  Operator=square
  Square1 : Math  Operator=square
  To Workspace : ToWorkspace  VariableName=ISE_ez  SaveFormat=Timeseries  SampleTime=-1
  To Workspace1 : ToWorkspace  VariableName=ISE_etheta  SaveFormat=Timeseries  SampleTime=-1
  To Workspace2 : ToWorkspace  VariableName=IAE_ez  SaveFormat=Timeseries  SampleTime=-1
  To Workspace3 : ToWorkspace  VariableName=IAE_etheta  SaveFormat=Timeseries  SampleTime=-1
  To Workspace4 : ToWorkspace  VariableName=ITAE_ez  SaveFormat=Timeseries  SampleTime=-1
  To Workspace5 : ToWorkspace  VariableName=ITAE_etheta  SaveFormat=Timeseries  SampleTime=-1
  To Workspace6 : ToWorkspace  VariableName=MSE_ez  SaveFormat=Timeseries  SampleTime=-1
  To Workspace7 : ToWorkspace  VariableName=MSE_etheta  SaveFormat=Timeseries  SampleTime=-1
  wires:
  zd/1 -> Add/1
  z_measured/1 -> Add/2
  theta_d/1 -> Add1/1
  theta_measured/1 -> Add1/2
  Add/1 -> Abs/1, Square/1
  Add1/1 -> Abs1/1, Square1/1
  Square/1 -> Integrator/1
  Square1/1 -> Integrator1/1
  Integrator/1 -> Divide/1, Scope2/1, Display/1, To Workspace/1
  Abs/1 -> Product/2, Integrator2/1
  Integrator2/1 -> Scope1/1, Display2/1, To Workspace2/1
  Integrator3/1 -> Scope4/1, Display3/1, To Workspace3/1
  Product/1 -> Integrator4/1
  Integrator4/1 -> Scope/1, Display4/1, To Workspace4/1
  Abs1/1 -> Integrator3/1, Product1/2
  Product1/1 -> Integrator5/1
  Integrator5/1 -> Scope3/1, To Workspace5/1, Display5/1
  Divide/1 -> To Workspace6/1, Display6/1, Scope6/1
  Divide1/1 -> Scope7/1, Display7/1, To Workspace7/1
  Max/1 -> Product/1, Divide1/2, Divide/2, Product1/1
  Integrator1/1 -> Divide1/1, Scope5/1, Display1/1, To Workspace1/1
  Constant/1 -> Max/2
  Clock/1 -> Max/1

== system Drone2_simulink_old1/Controller (STA-Based)/Subsystem1 ==
  note: RMS: Average Intensity and will reamin in N (newton)
  note: Integral of Square control : energy cost
  note: IAE: TOal fuel or Total Effort
  note: Smoothness: total variation
  force : Inport
  Abs : Abs  SaturateOnIntegerOverflow=off
  Abs1 : Abs  SaturateOnIntegerOverflow=off
  Discrete-Time Integrator : DiscreteIntegrator  IntegratorMethod=Accumulation: Backward Euler  gainval=0.001  SampleTime=-1  ICPrevOutput=DiscIntNeverNeededParam  ICPrevScaledInput=DiscIntNeverNeededParam
  Display{,1..4} (5 alike) : Display
  Integrator : Integrator
  Integrator1 : Integrator
  Integrator2 : Integrator
  RMS2 : dspstat3/RMS  run=off  directionMode=Each column  dimension=1  InputProcessing=Columns as channels (frame based)  reset_popup=None
  Scope{3..4,7..9} (5 alike) : Scope
  Square : Math  Operator=square
  Sum1 : Sum  Inputs=+-
  Unit Delay1 : UnitDelay  SampleTime=-1  HasFrameUpgradeWarning=on
  norm force : Subsystem
  Out Bus Element : Outport  PortName=Cost  Element=RMS
  Out Bus Element1 : Outport  PortName=Cost  Element=ISU
  Out Bus Element2 : Outport  PortName=Cost  Element=IAE
  Out Bus Element3 : Outport  PortName=Cost  Element=Smoothness
  wires:
  Sum1/1 -> Abs1/1
  force/1 -> norm force/1(force)
  norm force/1(sum) -> RMS2/1, Square/1, Abs/1
  Square/1 -> Integrator/1
  RMS2/1 -> Display/1, Out Bus Element/1, Scope3/1
  Unit Delay1/1 -> Sum1/2
  Abs/1 -> Integrator1/1, Sum1/1, Unit Delay1/1
  Integrator/1 -> Display1/1, Out Bus Element1/1, Scope4/1
  Integrator1/1 -> Display2/1, Scope7/1, Out Bus Element2/1
  Abs1/1 -> Discrete-Time Integrator/1, Integrator2/1
  Integrator2/1 -> Display4/1, Scope9/1
  Discrete-Time Integrator/1 -> Out Bus Element3/1, Scope8/1, Display3/1
